simulink model "velocity_subsystem_dob"  (R2019b)
settings: Solver=VariableStepAuto  StartTime=0.0  StopTime=20  RelTol=1e-3
values from neighbouring files (symbols this model uses):
  G__V_N_PX4 = G__q2_PX4_CL*(4*Tmax/m)*(1/s)    [dob_design.m]
  Q_2nd_DEM = [1 2*Q_zeta*wn wn^2]    [dob_design.m]
  Q_2nd_NUM = [0 0 1]    [dob_design.m]
undefined symbols (not defined in the file or in its folder): MPC_XY_VEL_D, MPC_XY_VEL_I, MPC_XY_VEL_P
libraries: simulink x2
settings Model: Creator=henry  LastModifiedBy=henry

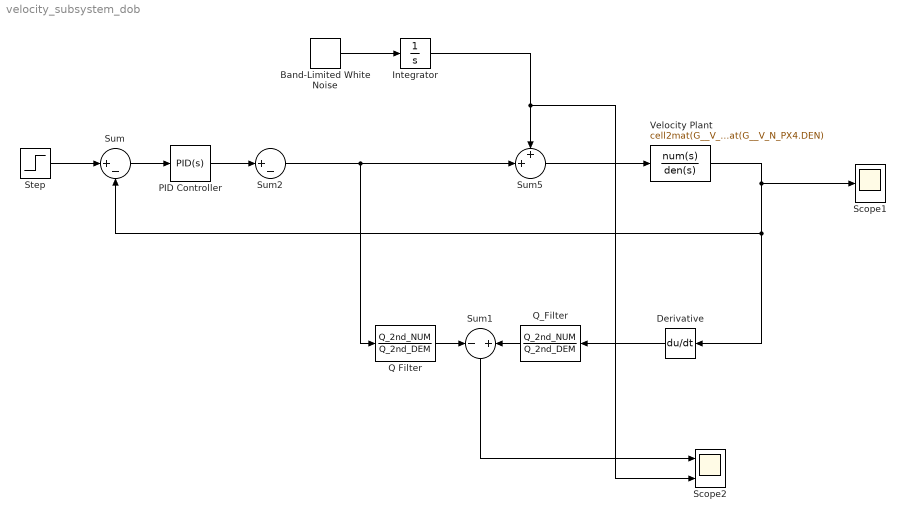
== system velocity_subsystem_dob ==
  Band-Limited White Noise : simulink/Sources/Band-Limited White Noise  Cov=[0.01]  Ts=0.1  seed=[23341]
  Derivative : Derivative
  Integrator : Integrator
  PID Controller : simulink/Continuous/PID Controller  Controller=PID  Form=Parallel  TimeDomain=Continuous-time  SampleTime=-1  IntegratorMethod=Forward Euler  FilterMethod=Forward Euler  ControllerParametersSource=internal  P=MPC_XY_VEL_P  I=MPC_XY_VEL_I  D=MPC_XY_VEL_D  UseFilter=on  N=100  TunerSelectOption=Transfer Function Based (PID Tuner App)  InitialConditionSource=internal  InitialConditionForIntegrator=0  InitialConditionForFilter=0  DifferentiatorICPrevScaledInput=0  ExternalReset=none  TrackingMode=off  Kt=1  LimitOutput=off  UpperSaturationLimit=inf  LowerSaturationLimit=-inf  LinearizeAsGain=on  AntiWindupMode=none  Kb=1  POutMin=[]  POutMax=[]  IOutMin=[]  IOutMax=[]  DOutMin=[]  DOutMax=[]  NOutMin=[]  NOutMax=[]  SumOutMin=[]  SumOutMax=[]  SaturationOutMin=[]  SaturationOutMax=[]  PParamMin=[]  PParamMax=[]  IParamMin=[]  IParamMax=[]  DParamMin=[]  DParamMax=[]  NParamMin=[]  NParamMax=[]  KbParamMin=[]  KbParamMax=[]  KtParamMin=[]  KtParamMax=[]  KbOutMin=[]  KbOutMax=[]  KtOutMin=[]  KtOutMax=[]  IntegratorOutMin=[]  IntegratorOutMax=[]  FilterOutMin=[]  FilterOutMax=[]  SumI1OutMin=[]  SumI1OutMax=[]  SumI2OutMin=[]  SumI2OutMax=[]  SumI3OutMin=[]  SumI3OutMax=[]  SumI4OutMin=[]  SumI4OutMax=[]  SumDOutMin=[]  SumDOutMax=[]  DifferentiatorOutMin=[]  DifferentiatorOutMax=[]  FilterDiffOutCoefMin=[]  FilterDiffOutCoefMax=[]  ReciprocalOutMin=[]  ReciprocalOutMax=[]  SumDenOutMin=[]  SumDenOutMax=[]  SumNumOutMin=[]  SumNumOutMax=[]  DivideOutMin=[]  DivideOutMax=[]  IntegratorContinuousStateAttributes=''  IntegratorStateMustResolveToSignalObject=off  IntegratorRTWStateStorageClass=Auto  FilterContinuousStateAttributes=''  FilterStateMustResolveToSignalObject=off  FilterRTWStateStorageClass=Auto  ParallelPVariant=InternalParameters  IdealPVariant=Disabled  IVariant=InternalParameters  DVariant=InternalParameters  IntegratorVariant=Continuous  SatVariant=Disabled  AWVariant=Passthrough  PCopyVariant=Disabled  TRVariant=Disabled  FdbkBlocksVariant=Forward  IdealPFdbkVariant=Disabled  SatFdbkVariant=Disabled  DerivativeFilterVariant=ContFilter  NVariant=InternalParameters  NCopyVariant=Disabled  FilterICVariant=InternalICsFilter  IntegratorICVariant=InternalICs  ExternalResetVariant=Disabled  TRSumVariant=Passthrough  SumFdbkVariant=Disabled  SumVariant=Sum_PID
  Q Filter : TransferFcn  Numerator=Q_2nd_NUM  Denominator=Q_2nd_DEM
  Q_Filter : TransferFcn  Numerator=Q_2nd_NUM  Denominator=Q_2nd_DEM
  Scope1 : Scope
  Scope2 : Scope  NumInputPorts=2
  Step : Step  Time=2  After=0  SampleTime=0
  Sum : Sum  Inputs=|+-
  Sum1 : Sum  Inputs=-+
  Sum2 : Sum  Inputs=|+-
  Sum5 : Sum  Inputs=++|
  Velocity Plant : TransferFcn  Numerator=cell2mat(G__V_N_PX4.NUM)  Denominator=cell2mat(G__V_N_PX4.DEN)
  wires:
  Velocity Plant/1 -> Scope1/1, Derivative/1, Sum/2
  Sum/1 -> PID Controller/1
  Step/1 -> Sum/1
  Sum5/1 -> Velocity Plant/1
  Q_Filter/1 -> Sum1/2
  Q Filter/1 -> Sum1/1
  PID Controller/1 -> Sum2/1
  Sum2/1 -> Q Filter/1, Sum5/2
  Derivative/1 -> Q_Filter/1
  Band-Limited White Noise/1 -> Integrator/1
  Sum1/1 -> Scope2/1
  Integrator/1 -> Scope2/2, Sum5/1
